simulink model "Constant2"  (Simulink 9.0)
settings: Solver=FixedStepAuto  StartTime=0.0  StopTime=10.0  FixedStep=0.1  RelTol=1e-3  EnableMultiTasking=on
settings Model: SuppressorTable=22 serialization::archive 11 0 6 0 0 0 0 0  Creator=arnaud  LastModifiedBy=hbourbou
settings DataIOCC: LimitDataPoints=on  SaveFormat=Structure  SignalLoggingSaveFormat=ModelDataLogs
settings OptimizationCC: ExpressionDepthLimit=2147483647
settings DebuggingCC: SolverPrmCheckMsg=warning  FcnCallInpInsideContextMsg=warning  StateNameClashWarn=warning  StrictBusMsg=Warning
settings GRTTargetCC: GeneratePreprocessorConditionals=Disable all  CombineOutputUpdateFcns=off  GRTInterface=on
settings ConfigComp: CovSFcnEnable=off

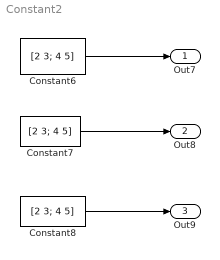
== system Constant2 ==
  Constant6 : Constant  Value=[2 3; 4 5]  OutDataTypeStr=double
  Constant7 : Constant  Value=[2 3; 4 5]  OutDataTypeStr=int8
  Constant8 : Constant  Value=[2 3; 4 5]  OutDataTypeStr=boolean
  Out7 : Outport
  Out8 : Outport  Port=2
  Out9 : Outport  Port=3
  wires:
  Constant6/1 -> Out7/1
  Constant7/1 -> Out8/1
  Constant8/1 -> Out9/1
